simulink model "Battlock_System2"  (R2025a)
settings: Solver=FixedStepDiscrete  StartTime=0.0  StopTime=10.0  FixedStep=0.01  RelTol=1e-3
libraries: simulink x1
settings Model: Creator=ishan  LastModifiedBy=HP

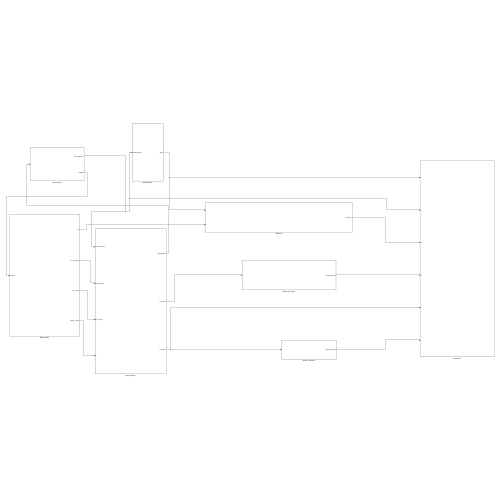
[thumbnail: Simulink's stored preview of the top-level diagram]
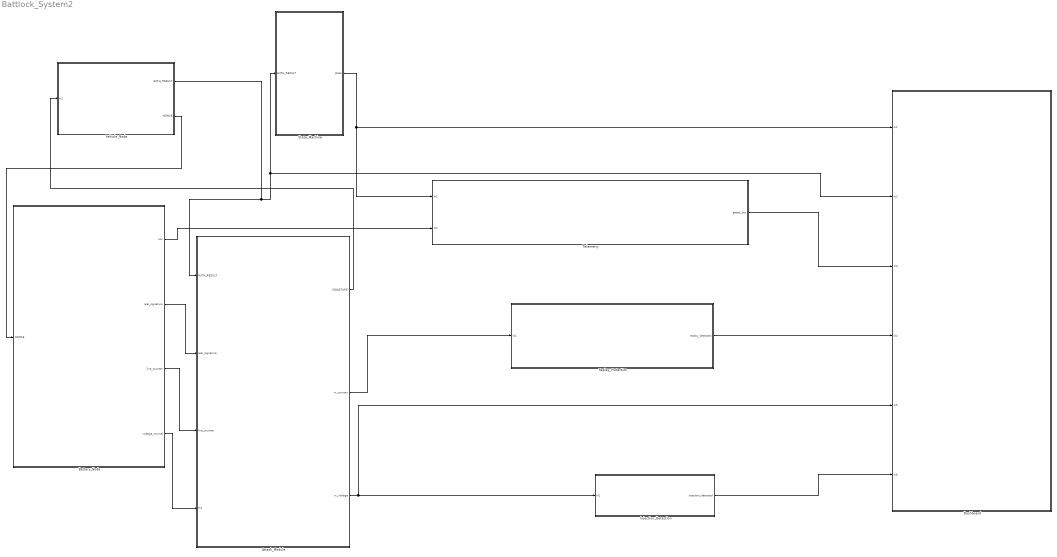
== system Battlock_System2 ==
  Attack_Module : Subsystem
  Battery_Node : Subsystem
  Dashboard : Subsystem
  Injection_Detection : Subsystem
  Replay_Protection : Subsystem
  State_Machine : Subsystem
  Telemetry : Subsystem
  Vehicle_Node : Subsystem
  wires:
  Attack_Module/3(rx_voltage) -> Dashboard/5(In5), Injection_Detection/1(In1)
  Attack_Module/2(rx_counter) -> Replay_Protection/1(In1)
  State_Machine/1(state) -> Telemetry/1(In1), Dashboard/1(In1)
  Battery_Node/2(real_signature) -> Attack_Module/2(real_signature)
  Battery_Node/3(live_counter) -> Attack_Module/3(live_counter)
  Battery_Node/4(voltage_normal) -> Attack_Module/4(In4)
  Vehicle_Node/1(AUTH_RESULT) -> State_Machine/1(AUTH_RESULT), Dashboard/2(In2), Attack_Module/1(AUTH_RESULT)
  Attack_Module/1(SIGNATURE) -> Vehicle_Node/1(In1)
  Vehicle_Node/2(NONCE) -> Battery_Node/1(NONCE)
  Battery_Node/1(soc) -> Telemetry/2(In2)
  Telemetry/1(gated_soc) -> Dashboard/3(In3)
  Replay_Protection/1(replay_detected) -> Dashboard/4(In4)
  Injection_Detection/1(injection_detected) -> Dashboard/6(In6)

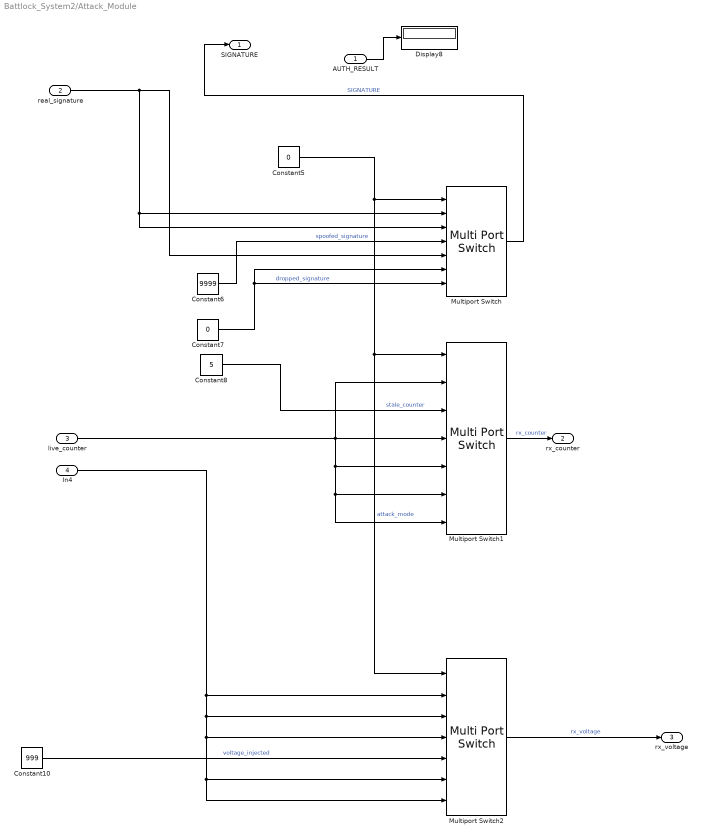
== system Battlock_System2/Attack_Module ==
  AUTH_RESULT : Inport
  real_signature : Inport  Port=2
  live_counter : Inport  Port=3
  In4 : Inport  Port=4
  Constant10 : Constant  Value=999
  Constant5 : Constant  Value=0
  Constant6 : Constant  Value=9999
  Constant7 : Constant  Value=0
  Constant8 : Constant  Value=5
  Display8 : Display
  Multiport Switch : MultiPortSwitch  DataPortOrder=Zero-based contiguous  Inputs=6  zeroidx=on  SaturateOnIntegerOverflow=off  InputSameDT=off
  Multiport Switch1 : MultiPortSwitch  DataPortOrder=Zero-based contiguous  Inputs=6  zeroidx=on  SaturateOnIntegerOverflow=off  InputSameDT=off
  Multiport Switch2 : MultiPortSwitch  DataPortOrder=Zero-based contiguous  Inputs=6  zeroidx=on  SaturateOnIntegerOverflow=off  InputSameDT=off
  SIGNATURE : Outport
  rx_counter : Outport  Port=2
  rx_voltage : Outport  Port=3
  wires:
  real_signature/1 -> Multiport Switch/3, Multiport Switch/2, Multiport Switch/5
  Constant10/1 -> Multiport Switch2/5  "voltage_injected"
  Constant5/1 -> Multiport Switch2/1, Multiport Switch1/1, Multiport Switch/1  "attack_mode"
  Constant6/1 -> Multiport Switch/4  "spoofed_signature"
  Constant7/1 -> Multiport Switch/6, Multiport Switch/7  "dropped_signature"
  live_counter/1 -> Multiport Switch1/7, Multiport Switch1/6, Multiport Switch1/5, Multiport Switch1/4, Multiport Switch1/2
  Constant8/1 -> Multiport Switch1/3  "stale_counter"
  Multiport Switch1/1 -> rx_counter/1  "rx_counter"
  AUTH_RESULT/1 -> Display8/1
  Multiport Switch/1 -> SIGNATURE/1  "SIGNATURE"
  Multiport Switch2/1 -> rx_voltage/1  "rx_voltage"
  In4/1 -> Multiport Switch2/7, Multiport Switch2/6, Multiport Switch2/4, Multiport Switch2/3, Multiport Switch2/2

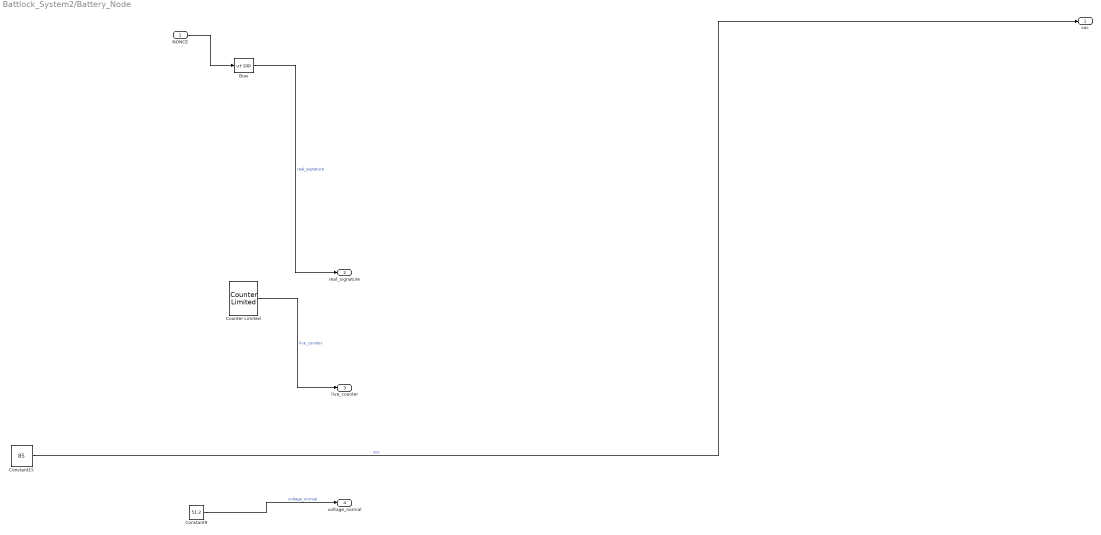
== system Battlock_System2/Battery_Node ==
  NONCE : Inport
  Bias : Bias  Bias=100  SaturateOnIntegerOverflow=off
  Constant15 : Constant  Value=85
  Constant9 : Constant  Value=51.2
  Counter Limited : simulink/Sources/Counter Limited  uplimit=255  tsamp=1
  soc : Outport
  real_signature : Outport  Port=2
  live_counter : Outport  Port=3
  voltage_normal : Outport  Port=4
  wires:
  Constant15/1 -> soc/1  "soc"
  Constant9/1 -> voltage_normal/1  "voltage_normal"
  NONCE/1 -> Bias/1
  Bias/1 -> real_signature/1  "real_signature"
  Counter Limited/1 -> live_counter/1  "live_counter"

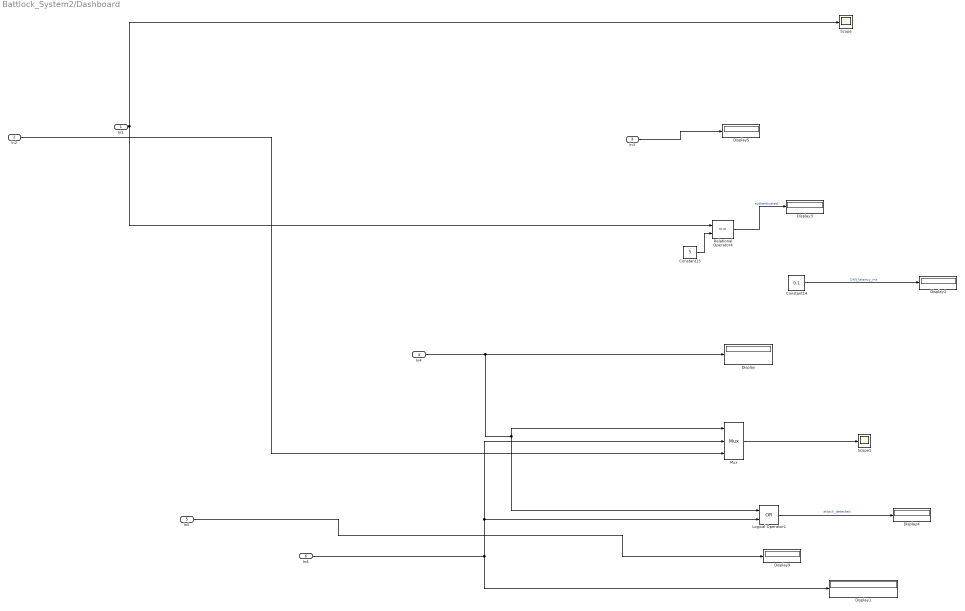
== system Battlock_System2/Dashboard ==
  In1 : Inport
  In2 : Inport  Port=2
  In3 : Inport  Port=3
  In4 : Inport  Port=4
  In5 : Inport  Port=5
  In6 : Inport  Port=6
  Constant13 : Constant  Value=5
  Constant14 : Constant  Value=0.1
  Display{,1..5,9} (7 alike) : Display
  Logical Operator1 : Logic  Operator=OR  AllPortsSameDT=off  OutDataTypeStr=boolean
  Mux : Mux  Inputs=3
  Relational Operator4 : RelationalOperator  Operator===  OutDataTypeStr=boolean  RndMeth=Simplest  InputSameDT=off
  Scope : Scope
      settings: ActiveDisplayYMinimum=-6.836402596325053  ActiveDisplayYMaximum=14.600813145765882
  Scope1 : Scope
      settings: ActiveDisplayYMinimum=-0.69242538567138889  ActiveDisplayYMaximum=1.664636042232656
  wires:
  In6/1 -> Mux/2, Logical Operator1/2, Display1/1
  In4/1 -> Display/1, Logical Operator1/1, Mux/1
  In2/1 -> Mux/3
  Logical Operator1/1 -> Display4/1  "attack_detected"
  Mux/1 -> Scope1/1
  Constant13/1 -> Relational Operator4/2
  Constant14/1 -> Display2/1  "CAN_latency_ms"
  Relational Operator4/1 -> Display3/1  "authenticated"
  In1/1 -> Scope/1, Relational Operator4/1
  In5/1 -> Display9/1
  In3/1 -> Display5/1

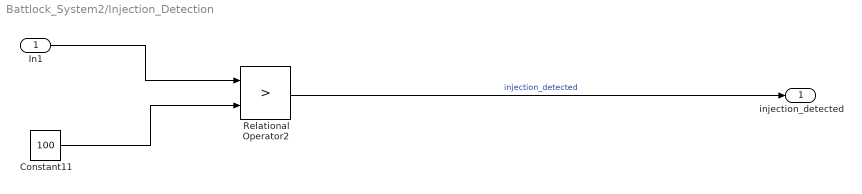
== system Battlock_System2/Injection_Detection ==
  In1 : Inport
  Constant11 : Constant  Value=100
  Relational Operator2 : RelationalOperator  Operator=>  OutDataTypeStr=boolean  RndMeth=Simplest  InputSameDT=off
  injection_detected : Outport
  wires:
  Constant11/1 -> Relational Operator2/2
  In1/1 -> Relational Operator2/1
  Relational Operator2/1 -> injection_detected/1  "injection_detected"

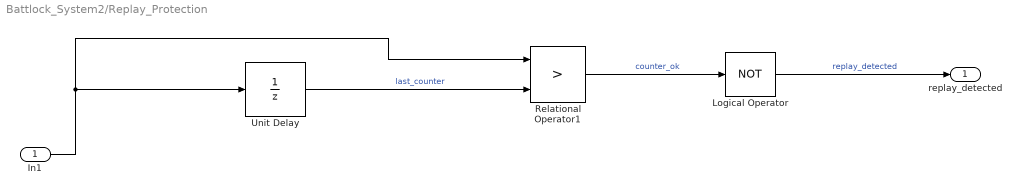
== system Battlock_System2/Replay_Protection ==
  In1 : Inport
  Logical Operator : Logic  Operator=NOT  AllPortsSameDT=off  OutDataTypeStr=boolean
  Relational Operator1 : RelationalOperator  Operator=>  OutDataTypeStr=boolean  RndMeth=Simplest  InputSameDT=off
  Unit Delay : UnitDelay  InitialCondition=-1  SampleTime=-1
  replay_detected : Outport
  wires:
  Relational Operator1/1 -> Logical Operator/1  "counter_ok"
  In1/1 -> Relational Operator1/1, Unit Delay/1
  Unit Delay/1 -> Relational Operator1/2  "last_counter"
  Logical Operator/1 -> replay_detected/1  "replay_detected"

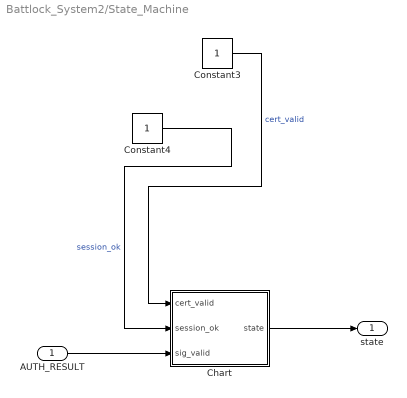
== system Battlock_System2/State_Machine ==
  AUTH_RESULT : Inport
  Chart : Stateflow chart  TreatAsAtomicUnit=on
  Constant3 : Constant
  Constant4 : Constant
  state : Outport
  wires:
  AUTH_RESULT/1 -> Chart/3(sig_valid)
  Constant3/1 -> Chart/1(cert_valid)  "cert_valid"
  Constant4/1 -> Chart/2(session_ok)  "session_ok"
  Chart/1(state) -> state/1

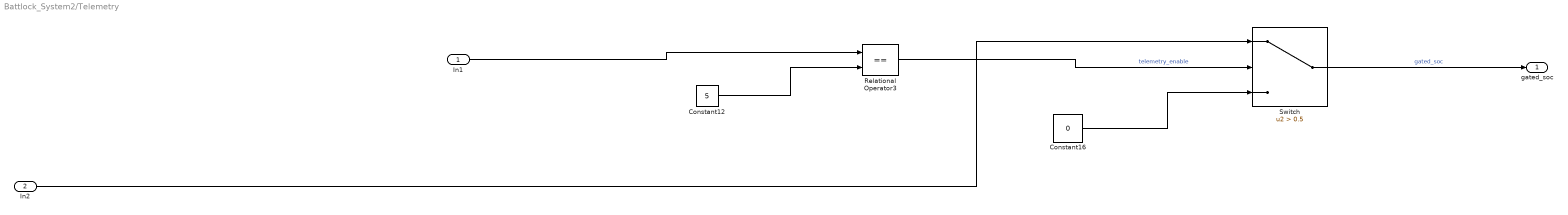
== system Battlock_System2/Telemetry ==
  In1 : Inport
  In2 : Inport  Port=2
  Constant12 : Constant  Value=5
  Constant16 : Constant  Value=0
  Relational Operator3 : RelationalOperator  Operator===  OutDataTypeStr=boolean  RndMeth=Simplest  InputSameDT=off
  Switch : Switch  Criteria=u2 > Threshold  Threshold=0.5  SaturateOnIntegerOverflow=off  InputSameDT=off
  gated_soc : Outport
  wires:
  Constant12/1 -> Relational Operator3/2
  Relational Operator3/1 -> Switch/2  "telemetry_enable"
  In1/1 -> Relational Operator3/1
  Constant16/1 -> Switch/3
  Switch/1 -> gated_soc/1  "gated_soc"
  In2/1 -> Switch/1

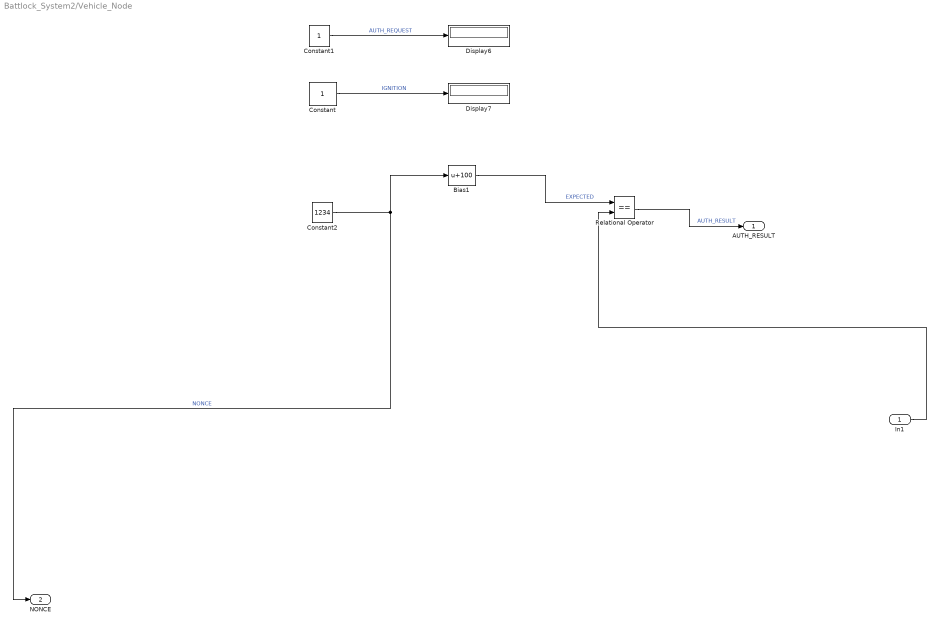
== system Battlock_System2/Vehicle_Node ==
  In1 : Inport
  Bias1 : Bias  Bias=100  SaturateOnIntegerOverflow=off
  Constant : Constant
  Constant1 : Constant
  Constant2 : Constant  Value=1234
  Display6 : Display
  Display7 : Display
  Relational Operator : RelationalOperator  Operator===  OutDataTypeStr=boolean  RndMeth=Simplest  InputSameDT=off
  AUTH_RESULT : Outport
  NONCE : Outport  Port=2
  wires:
  Constant2/1 -> NONCE/1, Bias1/1  "NONCE"
  Relational Operator/1 -> AUTH_RESULT/1  "AUTH_RESULT"
  Constant1/1 -> Display6/1  "AUTH_REQUEST"
  In1/1 -> Relational Operator/2
  Constant/1 -> Display7/1  "IGNITION"
  Bias1/1 -> Relational Operator/1  "EXPECTED"

== stateflow chart Battlock_System2/State_Machine/Chart ==
  state DISCONNECTED
    entry: state = 0;
  state HELLO_RECEIVED
    entry: state = 1;
  state CERT_VERIFIED
    entry: state = 2;
  state CHALLENGE_SENT
    entry: state = 3;
  state AUTHENTICATED
    entry: state = 4;
  state ACTIVE_SESSION
    entry: state = 5;
  (default) -> DISCONNECTED
  CHALLENGE_SENT -> DISCONNECTED [order 2] : after(1,sec)[~sig_valid]
  DISCONNECTED -> HELLO_RECEIVED : after(1,sec)
  HELLO_RECEIVED -> CERT_VERIFIED : after(1,sec)[cert_valid]
  CERT_VERIFIED -> CHALLENGE_SENT : after(1,sec)
  CHALLENGE_SENT -> AUTHENTICATED [order 1] : after(1,sec)[sig_valid]
  AUTHENTICATED -> ACTIVE_SESSION : after(1,sec)[session_ok]
  data: cert_valid input; session_ok input; sig_valid input; state output
